simulink model "Hanoi_OpenLoop_globals"  (R2014b)
settings: Solver=ode3  StartTime=0.0  StopTime=5  FixedStep=0.01  RelTol=1e-3
settings Model: Creator=lpark_000  LastModifiedBy=lpark_000

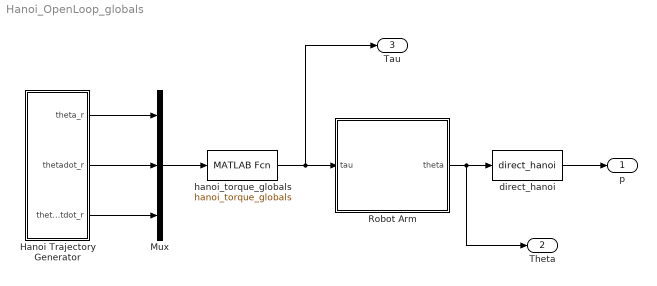
== system Hanoi_OpenLoop_globals ==
  Hanoi Trajectory Generator : Subsystem
  Mux : Mux  Inputs=3
  Robot Arm : Subsystem
  direct_hanoi : MATLABFcn  MATLABFcn=direct_hanoi
  hanoi_torque_globals : MATLABFcn  MATLABFcn=hanoi_torque_globals
  p : Outport
  Theta : Outport  Port=2
  Tau : Outport  Port=3
  wires:
  Robot Arm/1(theta) -> Theta/1, direct_hanoi/1
  direct_hanoi/1 -> p/1
  Hanoi Trajectory Generator/2(thetadot_r) -> Mux/2
  Hanoi Trajectory Generator/1(theta_r) -> Mux/1
  Hanoi Trajectory Generator/3(thetadotdot_r) -> Mux/3
  Mux/1 -> hanoi_torque_globals/1
  hanoi_torque_globals/1 -> Tau/1, Robot Arm/1(tau)

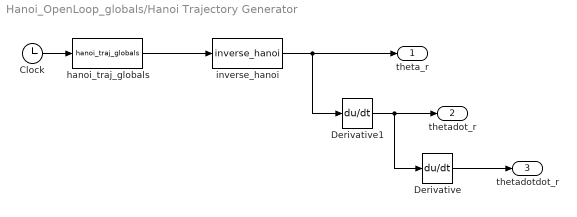
== system Hanoi_OpenLoop_globals/Hanoi Trajectory Generator ==
  Clock : Clock
  Derivative : Derivative
  Derivative1 : Derivative
  hanoi_traj_globals : MATLABFcn  MATLABFcn=hanoi_traj_globals
  inverse_hanoi : MATLABFcn  MATLABFcn=inverse_hanoi
  theta_r : Outport
  thetadot_r : Outport  Port=2
  thetadotdot_r : Outport  Port=3
  wires:
  Clock/1 -> hanoi_traj_globals/1
  inverse_hanoi/1 -> theta_r/1, Derivative1/1
  Derivative1/1 -> thetadot_r/1, Derivative/1
  Derivative/1 -> thetadotdot_r/1
  hanoi_traj_globals/1 -> inverse_hanoi/1

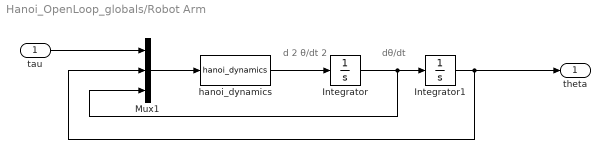
== system Hanoi_OpenLoop_globals/Robot Arm ==
  note: d 2 θ/dt 2
  note: dθ/dt
  tau : Inport
  Integrator : Integrator  InitialCondition=[0 0]
  Integrator1 : Integrator  InitialCondition=[pi/2, -pi/2]
  Mux1 : Mux  Inputs=3
  hanoi_dynamics : MATLABFcn  MATLABFcn=hanoi_dynamics
  theta : Outport
  wires:
  tau/1 -> Mux1/1
  Mux1/1 -> hanoi_dynamics/1
  Integrator/1 -> Mux1/3, Integrator1/1
  hanoi_dynamics/1 -> Integrator/1
  Integrator1/1 -> theta/1, Mux1/2
